simulink model "Subsystem"  (R2020b)
settings: Solver=VariableStepAuto  StartTime=0.0  StopTime=10.0  RelTol=1e-3
settings Model: Creator=Akshay A H  LastModifiedBy=Akshay A H
settings DataIOCC: SaveOutput=off  SaveTime=off

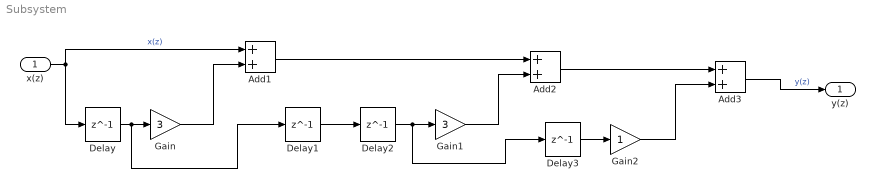
== system Subsystem ==
  x(z) : Inport  OutDataTypeStr=double  PortDimensions=1  SampleTime=0
  Add1 : Sum
  Add2 : Sum
  Add3 : Sum
  Delay{,1..3} (4 alike) : Delay  DelayLength=1
  Gain : Gain  Gain=3
  Gain1 : Gain  Gain=3
  Gain2 : Gain
  y(z) : Outport  OutDataTypeStr=double  PortDimensions=1  SampleTime=0
  wires:
  Delay2/1 -> Delay3/1, Gain1/1
  Add2/1 -> Add3/1
  Gain2/1 -> Add3/2
  Add1/1 -> Add2/1
  Delay1/1 -> Delay2/1
  Delay3/1 -> Gain2/1
  Gain1/1 -> Add2/2
  Delay/1 -> Gain/1, Delay1/1
  Gain/1 -> Add1/2
  x(z)/1 -> Add1/1, Delay/1  "x(z)"
  Add3/1 -> y(z)/1  "y(z)"
